simulink model "fullbridge1ph_mosfet_model2"  (R2026a)
settings: Solver=VariableStepAuto  StopTime=simStopTime
undefined symbols (not defined in the file): deadSamples, fout, fsw, ModIndex, Rload, Ts_ctrl, Vg
libraries: fl_lib x31, nesl_utility x28, ee_lib x11, simulink x1
settings Model: Creator=walmy  LastModifiedBy=walmy
settings SimscapeCC: SimscapeNominalValues="[{\"value\":\"1\",\"unit\":\"A\"},{\"value\":\"1\",\"unit\":\"bar\"},{\"value\":\"1\",\"unit\":\"cm^2\"},{\"value\":\"1\",\"unit\":\"cm^3/s\"},{\"value\":\"1\",\"unit\":\"kJ/kg\"},{\"value\":\"1\",\"unit\":\"kW\"},{\"value\":\"1\",\"unit\":\"l\"},{\"value\":\"1\",\"unit\":\"N\"},{\"value\":\"1\",\"unit\":\"N*m\"},{\"value\":\"1\",\"unit\":\"V\"}]"  SimscapeLogType=none  SimscapeLogDataHistory=5000.0

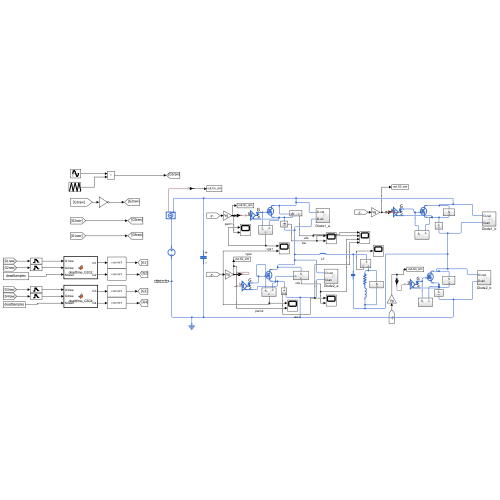
[thumbnail: Simulink's stored preview of the top-level diagram]
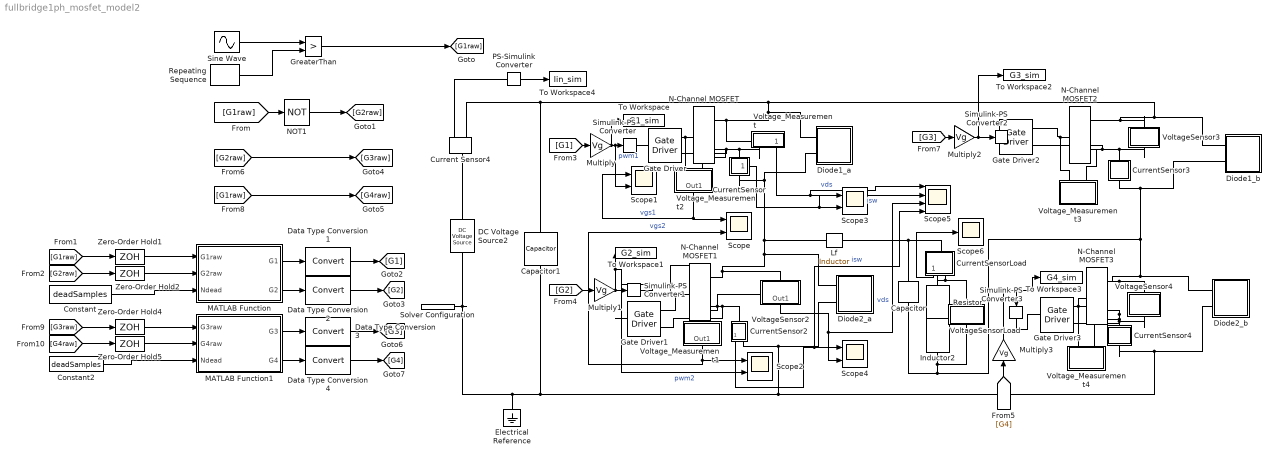
== system fullbridge1ph_mosfet_model2 ==
  Capacitor : fl_lib/Electrical/Electrical Elements/Capacitor  c=Cf F  r=0 Ohm  g=0 1/Ohm  i_specify=off  i_priority=None  i=0 A  i_nominal_specify=off  i_nominal_value=1  i_nominal_unit=A  v_specify=off  v_priority=High  v=0 V  v_nominal_specify=off  v_nominal_value=1  v_nominal_unit=V  vc_specify=on  vc_priority=High  vc=1 V  vc_nominal_specify=off  vc_nominal_value=1  vc_nominal_unit=V
  Capacitor1 : fl_lib/Electrical/Electrical Elements/Capacitor  c=Cdc F  r=0 Ohm  g=0 1/Ohm  i_specify=off  i_priority=None  i=0 A  i_nominal_specify=off  i_nominal_value=1  i_nominal_unit=A  v_specify=off  v_priority=High  v=Vdc V  v_nominal_specify=off  v_nominal_value=1  v_nominal_unit=V  vc_specify=on  vc_priority=High  vc=Vdc V  vc_nominal_specify=off  vc_nominal_value=1  vc_nominal_unit=V
  Constant : Constant  Value=deadSamples
  Constant2 : Constant  Value=deadSamples
  Current Sensor4 : fl_lib/Electrical/Electrical Sensors/Current Sensor
  CurrentSensor : Subsystem
      settings: PortSchema="{\"entries\":[{\"content\":{\"sides\":[{\"content\":{},\"type\":\"ConnectorPlacement.EquallySpacedRectSide\",\"uuid\":\"004a7a0d-f10a-4133-9832-9cba9dcbff9d\"},{\"content\":{\"connectorIds\":[\"Out1\"],\"side\":\"RIGHT\"},\"type\":\"ConnectorPlacement.EquallySpacedRectSide\",\"uuid\":\"56e408a5-c8db-4bda-b213-0e7e6169c543\"},{\"content\":{\"connectorIds\":[\"LConn1\"],\"side\":\"TOP\"},\"type\":\"ConnectorPlacement.EquallySpacedRectSide\",\"uuid\":\"d7e2417b-721d-4b46-aed4-551a16eadb47\"},{\"content\":{\"connectorIds\":[\"RConn1\"],\"side\":\"BOTTOM\"},\"type\":\"ConnectorPlacement.EquallySpacedRectSide\",\"uuid\":\"01b177b2-fa8e-4377-a3d9-543c30212534\"}]},\"type\":\"ConnectorPlacement.EquallySpacedConnector\",\"uuid\":\"4d702bd2-4ec5-4c77-8333-289479c4f2ec\"}],\"packageUris\":[\"http://schema.mathworks.com/mf0/Connector/R2020b\"],\"version\":\"1.0\"}"
  CurrentSensor2 : Subsystem
  CurrentSensor3 : Subsystem
  CurrentSensor4 : Subsystem
  CurrentSensorLoad : Subsystem
  DC Voltage Source2 : ee_lib/Additional Components/SPICE Sources/DC Voltage Source  DC=Vdc V
  Data Type Conversion{1..4} (4 alike) : DataTypeConversion  SaturateOnIntegerOverflow=off  RndMeth=Floor
  Diode1_a : Subsystem
  Diode1_b : Subsystem
  Diode2_a : Subsystem
  Diode2_b : Subsystem
  Electrical Reference : fl_lib/Electrical/Electrical Elements/Electrical Reference
  Gate Driver{,1..3} (4 alike) : ee_lib/Semiconductors & Converters/Gate Driver  port_option=ee.enum.controlport.ps  uHigh=2.0 V  uLow=0.8 V  uHighValue=0.7  uLowValue=0.3  vHigh=Vg V  vLow=-Vg V  tHigh=50 ns  tLow=50 ns  parameterization=ee.enum.semiconductors.gateDriverParam.outputImpedance  rHigh=Rg_on Ohm  rLow=Rg_off Ohm  tRise=20 ns  tFall=20 ns  cLoad=10 nF  ZonTime_specify=off  ZonTime_priority=None  ZonTime=0 s  ZoffTime_specify=off  ZoffTime_priority=None  ZoffTime=0 s
  GreaterThan : RelationalOperator  Operator=>  OutDataTypeStr=boolean  RndMeth=Simplest  InputSameDT=off
  Inductor2 : ee_lib/Passive/Inductor  l=Lload H  enable_L_tol=ee.enum.toleranceApplication.none  L_tol=20  tol_distribution=ee.enum.toleranceDistribution.uniform  nSigma=4  r=0 Ohm  g=1e-9 1/Ohm  enable_operating_limits=ee.enum.enable.no  operating_limit_action=ee.enum.passive.reportOpLim.warn  max_working_current=1 A  power_rating=1 W  i_L_specify=on  i_L_priority=Low  i_L=0 A  i_L_nominal_specify=off  i_L_nominal_value=1  i_L_nominal_unit=A
  Lf : ee_lib/Passive/Inductor  l=Lf H  enable_L_tol=ee.enum.toleranceApplication.none  L_tol=20  tol_distribution=ee.enum.toleranceDistribution.uniform  nSigma=4  r=0 Ohm  g=1e-9 1/Ohm  enable_operating_limits=ee.enum.enable.no  operating_limit_action=ee.enum.passive.reportOpLim.warn  max_working_current=1 A  power_rating=1 W  i_L_specify=on  i_L_priority=Low  i_L=0 A  i_L_nominal_specify=off  i_L_nominal_value=1  i_L_nominal_unit=A
  MATLAB Function : MATLAB Function  TreatAsAtomicUnit=on
  MATLAB Function1 : MATLAB Function  TreatAsAtomicUnit=on
  Multiply{,1..3} (4 alike) : Gain  Gain=Vg
  N-Channel MOSFET{,1..3} (4 alike) : ee_lib/Semiconductors & Converters/N-Channel MOSFET  paramTerminal=ee.enum.mosfet.numberOfTerminals.three  parameterization=ee.enum.mosfet.parameterization.datasheet  Beta=5.0 A/V^2  Rds=RdsOn Ohm  Id=Ids_RdsOn A  Vgs=Vgs_RdsOn V  Vth=Vth_sw V  Vth0=1.7 V  lam=0 1/V  gamma_vth=0.5 V^(1/2)  phib=0.5 V  Vth1=1.9071 V  Vbs1=-1 V  Vth2=2.066 V  Vbs2=-2 V  Tmeas=25 degC  Vgs_vec=[-1, -.5, 2, 3, 4, 5] V  Vds_vec=[0, 2, 4, 8, 12, 16, 20] V  Vbs_vec=[0, -4, -6, -12] V  T_vec=[25, 125] degC  Vth_vec=[.4, 1.2, 1.4, 1.45] V  Vth_mat=[.4, .35; 1.2, 1.15; 1.4, 1.35; 1.45, 1.4] V  Ids_mat=[0, 0, 0, 0, 0, 0, 0; 0, 0, 0, 0, 0, 0, 0; 0, .003, .0038, .0043, .0046, .0048, .0049; 0, .0055, .008, .009, .0095, .01, .0101; 0, .0115, .016, .018, .019, .0195, .02; 0, .0152, .0225, .0265, .028, .0295, .03] A  Ids_mat0=[0, 0, 0, 0, 0, 0, 0; 0, 0, 0, 0, 0, 0, 0; 0, .003, .0038, .0043, .0046, .0048, .0049; 0, .0055, .008, .009, .0095, .01, .0101; 0, .0115, .016, .018, .019, .0195, .02; 0, .0152, .0225, .0265, .028, .0295, .03] A  Ids_mat_3D=zeros(6, 7, 2) A  Ids_mat_3D0=zeros(6, 7, 2) A  IV_table_symmetry=ee.enum.mosfet.symmetricNIV.no  RS=0 Ohm  RD=0 Ohm  RB=0.001 Ohm  LeadRs=0 Ohm  LeadRd=0 Ohm  LeadRg=0 Ohm  LeadRb=0 Ohm  LS=0 nH  LD=0 nH  LG=0 nH  LB=0 nH  C_param=ee.enum.mosfet.capacitanceParam.fixedciss  C_GS=270 pF  C_GD=80 pF  C_GB=0 pF  C_DS=0 pF  C_iss=Ciss_sw_pF pF  C_rss=Crss_sw_pF pF  C_oss=Coss_sw_pF pF  C_iss_vec=[720, 700, 590, 470, 390, 310] pF  C_rss_vec=[450, 400, 300, 190, 95, 55] pF  C_oss_vec=[900, 810, 690, 420, 270, 170] pF  C_GS_vec=[270, 300, 290, 280, 295, 255] pF  C_GD_vec=[450, 400, 300, 190, 95, 55] pF  C_GB_vec=[270, 300, 290, 280, 295, 255] pF  C_Vgs_vec=0 V  C_DS_vec=[450, 410, 390, 230, 175, 115] pF  C_Vds_vec=[.1, .3, 1, 3, 10, 30] V  V_GS_for_cap_data=0 V  charge_linearity_param=ee.enum.mosfet.cgdLinearity.constant  C_OX=200 pF  V_C_OX=-0.5 V  charge_linearity_param_vgb=ee.enum.mosfet.cgbLinearity.instantly  charge_linearity_param_with_vgb=ee.enum.mosfet.cgbLinearityWithSeparateCgb.instantly  Di_param=ee.enum.mosfet.diodeParam.no  IsDiode=BodyDiodeIs A  Vbi=BodyDiodeVbi V  n=BodyDiodeN  Cj0Diode=BodyDiodeCj F  TT=BodyDiodeTT s  Tmeas_dio=25 degC  TableTypeNoT=ee.enum.mosfet.tableType.IfMat  TableType=ee.enum.diode.tableType.IfMat  IfVec=[.07, .12, .19, 1.75, 4.24, 7.32, 11.2] A  IfMat=[.07, .12, .19, 1.75, 4.24, 7.32, 11.2; .16, .3, .72, 2.14, 4.02, 6.35, 9.12] A  VfVecV=[.9, 1.15, 1.25, 1.5, 1.75, 2.17, 2.6, 2.85] V  VfMatV=[.9, 1.15, 1.25, 1.5, 1.75, 2.17, 2.6, 2.85; .58, .68, .75, 1.1, 1.38, 1.77, 2.27, 2.7] V  TjVec=[25, 125] degC  VfVec=[.5, .7, .9, 1.3, 1.7, 2.1, 2.5] V  IfVecV=[.1, .2, .5, 1, 2, 4, 7, 10] A  diode_Goff=1e-12 1/Ohm  prmDatasheet=ee.enum.temperatureParameterization.none  prmEquCoeff=ee.enum.temperatureParameterization.none  dVth_dT=-6 mV/K  dVth0_dT=-6 mV/K  Rds_T2=0.037 Ohm  BEXDatasheet=-1.5  BEXEquCoeff=-1.5  etaisDatasheet=3  etaisEquCoeff=3  Tmeas2=125 degC  etaisTabulated=3  TdeviceDatasheet=25 degC  TdeviceEquCoeff=25 degC  TdeviceTabulated=25 degC  i_g_specify=off  i_g_priority=None  i_g=0 A  i_g_nominal_specify=off  i_g_nominal_value=1  i_g_nominal_unit=A  i_d_specify=off  i_d_priority=None  i_d=0 A  i_d_nominal_specify=off  i_d_nominal_value=1  i_d_nominal_unit=A  i_b_specify=off  i_b_priority=None  i_b=0 A  i_b_nominal_specify=off  i_b_nominal_value=1  i_b_nominal_unit=A  voltage_gs_specify=off  voltage_gs_priority=None  voltage_gs=0 V  voltage_gs_nominal_specify=off  voltage_gs_nominal_value=1  voltage_gs_nominal_unit=V  voltage_ds_specify=off  voltage_ds_priority=None  voltage_ds=0 V  voltage_ds_nominal_specify=off  voltage_ds_nominal_value=1  voltage_ds_nominal_unit=V  voltage_bs_specify=off  voltage_bs_priority=None  voltage_bs=0 V  voltage_bs_nominal_specify=off  voltage_bs_nominal_value=1  voltage_bs_nominal_unit=V  v_Cgs_specify=off  v_Cgs_priority=High  v_Cgs=0 V  v_Cgs_nominal_specify=off  v_Cgs_nominal_value=1  v_Cgs_nominal_unit=V  v_Cds_specify=on  v_Cds_priority=Low  v_Cds=0 V  v_Cds_nominal_specify=off  v_Cds_nominal_value=1  v_Cds_nominal_unit=V  v_Cbs_specify=off  v_Cbs_priority=High  v_Cbs=0 V  v_Cbs_nominal_specify=off  v_Cbs_nominal_value=1  v_Cbs_nominal_unit=V  thermal_network_parameterization=ee.enum.thermalNetworkTopology.junctionCase  Rth=[0, 10] K/W  Rth_Cauer=[1, 3, 10] K/W  Rth_Foster=[.08, .14, .22, .16] K/W  thermal_mass_parameterization=ee.enum.thermalNetwork.timeconstant  thermal_mass=[0, 1] J/K  thermal_mass_Cauer=[.1, .3, 1] J/K  thermal_mass_Foster=[.001, .005, .05, .5] J/K  thermal_time_constant=[0, 10] s  thermal_time_constant_Cauer=[1, 3, 10] s  thermal_time_constant_Foster=[7e-05, .0007, .01, .08] s  thermal_mass_initial_temperatures=[25, 25] degC  thermal_mass_initial_temperatures_Cauer=[25, 25, 25] degC  Tvec_initial_Foster=[25, 25, 25, 25] degC  betaref=18 A/V^2  Vfbref=-1.1 V  gamma=3.5 V^(1/2)  phib2ref=1 V  thesatref=0.4 1/V  alpha=0  Vp=5e-2 V  thesrref=0 1/V  m=8  Tref=25 degC  Rsref=2e-3 Ohm  Rdref=0.17 Ohm  Rgref=8.4 Ohm  Rbref=2e-3 Ohm  Cox=1500 pF  Cgso=100 pF  Cgdo=14 pF  Isref=5.2e-13 A  Cj0=480 pF  Tprm=ee.enum.temperatureParameterization.none  etabet=1.3  Stvfb=5e-4 V/K  Stphib=-8.5e-4 V/K  etasat=1.04  etasr=0.65  etar=0.95  etais=3  Tsim=25 degC  Ig_specify=off  Ig_priority=None  Ig=0 A  Ig_nominal_specify=off  Ig_nominal_value=1  Ig_nominal_unit=nA  Ids_specify=off  Ids_priority=None  Ids=0 A  Ids_nominal_specify=off  Ids_nominal_value=1  Ids_nominal_unit=A  Ib_specify=off  Ib_priority=None  Ib=0 A  Ib_nominal_specify=off  Ib_nominal_value=1  Ib_nominal_unit=uA  V_gs_specify=off  V_gs_priority=None  V_gs=0 V  V_gs_nominal_specify=off  V_gs_nominal_value=1  V_gs_nominal_unit=V  V_ds_specify=off  V_ds_priority=None  V_ds=0 V  V_ds_nominal_specify=off  V_ds_nominal_value=1  V_ds_nominal_unit=V  V_bs_specify=off  V_bs_priority=None  V_bs=0 V  V_bs_nominal_specify=off  V_bs_nominal_value=1  V_bs_nominal_unit=V  QGoverCox_specify=off  QGoverCox_priority=None  QGoverCox=0 V  QGoverCox_nominal_specify=off  QGoverCox_nominal_value=1  QGoverCox_nominal_unit=V  QDoverCox_specify=off  QDoverCox_priority=None  QDoverCox=0 V  QDoverCox_nominal_specify=off  QDoverCox_nominal_value=1  QDoverCox_nominal_unit=V  QBoverCox_specify=off  QBoverCox_priority=None  QBoverCox=0 V  QBoverCox_nominal_specify=off  QBoverCox_nominal_value=1  QBoverCox_nominal_unit=V  T0=[25, 25] degC  T0_Cauer=[25, 25, 25] degC
  NOT1 : Logic  Operator=NOT  IconShape=distinctive  AllPortsSameDT=off  OutDataTypeStr=boolean
  PS-Simulink Converter : nesl_utility/PS-Simulink Converter  PhysicalDomain=network_engine_domain  SubClassName=ps_output  LeftPortType=input  RightPortType=output  PseudoPeriodic=off  Frequencies=[]  VectorFormat=inherit  Unit=inherit  AffineConversion=off
  Repeating Sequence : simulink/Sources/Repeating Sequence  rep_seq_t=[0 1/(2*fsw) 1/fsw]  rep_seq_y=[-1 1 -1]
  Resistor : fl_lib/Electrical/Electrical Elements/Resistor  R=Rload Ohm  i_specify=off  i_priority=None  i=0 A  i_nominal_specify=off  i_nominal_value=1  i_nominal_unit=A  v_specify=off  v_priority=None  v=0 V  v_nominal_specify=off  v_nominal_value=1  v_nominal_unit=V
  Scope{,1..4} (5 alike) : Scope  NumInputPorts=2
      Scope settings: ActiveDisplayYMinimum=-1.8442714573243091  ActiveDisplayYMaximum=11.329599284020166  DataLoggingVariableName=ScopeData2
      Scope1 settings: ActiveDisplayYMinimum=-1.6421747300623222  ActiveDisplayYMaximum=11.343693671801418  DataLoggingVariableName=ScopeData3
      Scope2 settings: ActiveDisplayYMinimum=-1  ActiveDisplayYMaximum=1  DataLoggingVariableName=ScopeData4
      Scope3 settings: ActiveDisplayYMinimum=-18.171152475957115  ActiveDisplayYMaximum=421.06855498709  DataLoggingVariableName=ScopeData5
      Scope4 settings: ActiveDisplayYMinimum=-1  ActiveDisplayYMaximum=1  DataLoggingVariableName=ScopeData6
  Scope5 : Scope  NumInputPorts=4
      settings: ActiveDisplayYMinimum=-77.946677692025617  ActiveDisplayYMaximum=455.393739095461  DataLoggingVariableName=ScopeData7
  Scope6 : Scope
      settings: ActiveDisplayYMinimum=-11.968033507226483  ActiveDisplayYMaximum=12.230491562923556
  Simulink-PS Converter{,1..3} (4 alike) : nesl_utility/Simulink-PS Converter  PhysicalDomain=network_engine_domain  SubClassName=ps_input  LeftPortType=input  RightPortType=output  PseudoPeriodic=off  Frequencies=[]  NoiseDistribution=none  NoiseParameters=[]  Unit=1  AffineConversion=off  FilteringAndDerivatives=provide  SimscapeFilterOrder=1  InputFilterTimeConstant=0.001  UdotUserProvided=0
  Sine Wave : Sin  Amplitude=ModIndex  Frequency=2*pi*fout  SampleTime=0
  Solver Configuration : nesl_utility/Solver Configuration  PhysicalDomain=network_engine_domain  SubClassName=solver  LeftPortType=input  RightPortType=generic  Tones=[]  Harmonics=[]  SimulateNoise=off  Profile=off  UseLocalSampling=off  EnableSwitchedLinearOptims=on  FrequencyDomain=off  UseCCode=off  RelTol=0.001  AbsTol=0.001  MinStep=1e-09  ToWorkspace=off  RevertToSquareIcSolve=off  NumHomotopyIterations=100  PhasorMode=off  PhasorModeNumHarmonics=1  ConsistencySolver=NEWTON_XTOL_AFTER_FTOL  CanonicalOrdering=UNORDERED  OptimizeIntermediates=UNOPTIMIZED  IndexReductionMethod=DerivativeReplacement  DoDC=off  ResidualTolerance=1e-09  ConsistencyTolSource=GLOBAL  ConsistencyAbsTol=0.001  ConsistencyRelTol=0.001  ConsistencyTolFactor=0.001  UseLocalSolver=on  LocalSolverChoice=NE_BACKWARD_EULER_ADVANCER  ResolveIndetEquations=on  FunctionEvalNumThread=1  LocalSolverSampleTime=50e-09  DoFixedCost=off  MaxNonlinIter=3  MaxModeIter=2  ComputeImpulses=off  ImpulseIterations=2  LinearAlgebra=auto  LinearAlgebraNumThread=0  EquationFormulation=NE_TIME_EF  DelaysMemoryBudget=1024  AutomaticFiltering=on  FilteringTimeConstant=0.001  PartitionStorageMethod=AS_NEEDED  PartitionMemoryBudget=1024  PartitionMethod=ROBUST  MultibodyUseLocalSolver=off  MultibodyLocalSolverChoice=ODE1  MultibodyLocalSolverSampleTime=0.001
  To Workspace : ToWorkspace  VariableName=G1_sim  SaveFormat=Timeseries  SampleTime=-1
  To Workspace1 : ToWorkspace  VariableName=G2_sim  SaveFormat=Timeseries  SampleTime=-1
  To Workspace2 : ToWorkspace  VariableName=G3_sim  SaveFormat=Timeseries  SampleTime=-1
  To Workspace3 : ToWorkspace  VariableName=G4_sim  SaveFormat=Timeseries  SampleTime=-1
  To Workspace4 : ToWorkspace  VariableName=Iin_sim  SaveFormat=Timeseries  SampleTime=-1
  VoltageSensor2 : Subsystem
      settings: PortSchema="{\"entries\":[{\"content\":{\"sides\":[{\"content\":{\"connectorIds\":[\"LConn1\"]},\"type\":\"ConnectorPlacement.EquallySpacedRectSide\",\"uuid\":\"21f317c2-e9e3-4775-bc2b-f44589605b73\"},{\"content\":{\"connectorIds\":[\"Out1\"],\"side\":\"RIGHT\"},\"type\":\"ConnectorPlacement.EquallySpacedRectSide\",\"uuid\":\"b0a4b85f-57a9-4dd8-a5ef-f426b86bae19\"},{\"content\":{\"connectorIds\":[\"LConn2\"],\"side\":\"TOP\"},\"type\":\"ConnectorPlacement.EquallySpacedRectSide\",\"uuid\":\"154dd31c-2e34-446c-ad4e-468f30782d57\"}]},\"type\":\"ConnectorPlacement.EquallySpacedConnector\",\"uuid\":\"ce3d8c78-d9da-4da1-88e6-92c14a3c1d9d\"}],\"packageUris\":[\"http://schema.mathworks.com/mf0/Connector/R2020b\"],\"version\":\"1.0\"}"
  VoltageSensor3 : Subsystem
  VoltageSensor4 : Subsystem
  VoltageSensorLoad : Subsystem
  Voltage_Measurement : Subsystem
      settings: PortSchema="{\"entries\":[{\"content\":{\"sides\":[{\"content\":{},\"type\":\"ConnectorPlacement.EquallySpacedRectSide\",\"uuid\":\"05335a37-bb92-4dc1-a41e-097329ec8732\"},{\"content\":{\"connectorIds\":[\"RConn1\",\"Out1\"],\"side\":\"RIGHT\"},\"type\":\"ConnectorPlacement.EquallySpacedRectSide\",\"uuid\":\"ddc17991-7e8e-4870-a1a0-8b769323db05\"},{\"content\":{\"connectorIds\":[\"LConn1\"],\"side\":\"TOP\"},\"type\":\"ConnectorPlacement.EquallySpacedRectSide\",\"uuid\":\"7075b36f-b4e1-42ca-a61e-d199b225f25e\"}]},\"type\":\"ConnectorPlacement.EquallySpacedConnector\",\"uuid\":\"382df35e-8f74-4d81-944e-45ad513cff4b\"}],\"packageUris\":[\"http://schema.mathworks.com/mf0/Connector/R2020b\"],\"version\":\"1.0\"}"
  Voltage_Measurement1 : Subsystem
  Voltage_Measurement2 : Subsystem
  Voltage_Measurement3 : Subsystem
  Voltage_Measurement4 : Subsystem
  Zero-Order Hold{1..2,4..5} (4 alike) : ZeroOrderHold  SampleTime=Ts_ctrl
  wires:
  [G1raw] -> Zero-Order Hold1/1
  [G2raw] -> Zero-Order Hold2/1
  MATLAB Function/1(G1) -> Data Type Conversion1/1
  MATLAB Function/2(G2) -> Data Type Conversion2/1
  [G1] -> Multiply/1
  Multiply3/1 -> To Workspace3/1, Simulink-PS Converter3/1
  Multiply2/1 -> To Workspace2/1, Simulink-PS Converter2/1
  [G1raw] -> NOT1/1
  NOT1/1 -> [G2raw]
  GreaterThan/1 -> [G1raw]
  Sine Wave/1 -> GreaterThan/1
  Repeating Sequence/1 -> GreaterThan/2
  [G2] -> Multiply1/1
  [G3] -> Multiply2/1
  [G4] -> Multiply3/1
  Data Type Conversion1/1 -> [G1]
  Data Type Conversion2/1 -> [G2]
  [G2raw] -> [G3raw]
  [G1raw] -> [G4raw]
  Data Type Conversion4/1 -> [G4]
  Data Type Conversion3/1 -> [G3]
  MATLAB Function1/2(G4) -> Data Type Conversion4/1
  MATLAB Function1/1(G3) -> Data Type Conversion3/1
  Constant2/1 -> MATLAB Function1/3(Ndead)
  [G4raw] -> Zero-Order Hold5/1
  [G3raw] -> Zero-Order Hold4/1
  Multiply1/1 -> Scope2/2, To Workspace1/1, Simulink-PS Converter1/1  "pwm2"
  Multiply/1 -> To Workspace/1, Simulink-PS Converter/1, Scope1/2  "pwm1"
  Voltage_Measurement2/1(Out1) -> Scope/1, Scope1/1  "vgs1"
  Voltage_Measurement1/1(Out1) -> Scope2/1, Scope/2  "vgs2"
  Voltage_Measurement/1(Out1) -> Scope5/1, Scope3/1  "vds"
  CurrentSensor/1(Out1) -> Scope5/2, Scope3/2  "isw"
  CurrentSensor2/1(Out1) -> Scope5/4, Scope4/1  "isw"
  VoltageSensor2/1(Out1) -> Scope5/3, Scope4/2  "vds"
  CurrentSensorLoad/1(Out1) -> Scope6/1
  PS-Simulink Converter/1 -> To Workspace4/1
  Zero-Order Hold1/1 -> MATLAB Function/1(G1raw)
  Zero-Order Hold2/1 -> MATLAB Function/2(G2raw)
  Constant/1 -> MATLAB Function/3(Ndead)
  Zero-Order Hold4/1 -> MATLAB Function1/1(G3raw)
  Zero-Order Hold5/1 -> MATLAB Function1/2(G4raw)
  connections:
  CurrentSensor4/RConn1 -- Solver Configuration/RConn1 -- DC Voltage Source2/RConn1 -- Electrical Reference/LConn1 -- Capacitor1/RConn1 -- Diode2_a/LConn2 -- CurrentSensor2/RConn1 -- Diode2_b/LConn2
  Diode1_a/LConn1 -- Voltage_Measurement/LConn1 -- N-Channel MOSFET/RConn1 -- Current Sensor4/RConn2 -- Capacitor1/LConn1 -- VoltageSensor3/LConn1 -- N-Channel MOSFET2/RConn1 -- Diode1_b/LConn1
  N-Channel MOSFET/RConn2 -- Voltage_Measurement/RConn1 -- CurrentSensor/LConn1 -- Gate Driver/RConn2 -- Voltage_Measurement2/LConn2
  CurrentSensor2/LConn1 -- Voltage_Measurement1/LConn2 -- VoltageSensor2/LConn2 -- Gate Driver1/RConn2 -- N-Channel MOSFET1/RConn2
  Diode2_a/LConn1 -- Diode1_a/LConn2 -- CurrentSensor/RConn1 -- Lf/LConn1 -- VoltageSensor2/LConn1 -- N-Channel MOSFET1/RConn1
  CurrentSensor3/LConn1 -- Voltage_Measurement3/LConn2 -- Gate Driver2/RConn2 -- N-Channel MOSFET2/RConn2 -- VoltageSensor3/RConn1
  Inductor2/RConn1 -- CurrentSensor3/RConn1 -- Diode1_b/LConn2 -- VoltageSensor4/LConn1 -- N-Channel MOSFET3/RConn1 -- Diode2_b/LConn1 -- Capacitor/RConn1 -- VoltageSensorLoad/RConn1
  CurrentSensor4/LConn1 -- Gate Driver3/RConn2 -- VoltageSensor4/RConn1 -- Voltage_Measurement4/LConn2 -- N-Channel MOSFET3/RConn2
  Capacitor/LConn1 -- CurrentSensorLoad/LConn1 -- Lf/RConn1
  Resistor/LConn1 -- VoltageSensorLoad/LConn1 -- CurrentSensorLoad/RConn1
  Resistor/RConn1 -- Inductor2/LConn1
  Gate Driver/RConn1 -- Voltage_Measurement2/LConn1 -- N-Channel MOSFET/LConn1
  Simulink-PS Converter/RConn1 -- Gate Driver/LConn1
  Gate Driver1/LConn1 -- Simulink-PS Converter1/RConn1
  Gate Driver2/LConn1 -- Simulink-PS Converter2/RConn1
  Voltage_Measurement3/LConn1 -- Gate Driver2/RConn1 -- N-Channel MOSFET2/LConn1
  Simulink-PS Converter3/RConn1 -- Gate Driver3/LConn1
  Gate Driver3/RConn1 -- Voltage_Measurement4/LConn1 -- N-Channel MOSFET3/LConn1
  Current Sensor4/LConn1 -- DC Voltage Source2/LConn1
  PS-Simulink Converter/LConn1 -- Current Sensor4/RConn1
  Gate Driver1/RConn1 -- Voltage_Measurement1/LConn1 -- N-Channel MOSFET1/LConn1

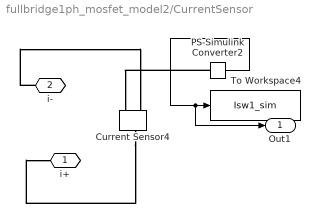
== system fullbridge1ph_mosfet_model2/CurrentSensor ==
  Current Sensor4 : fl_lib/Electrical/Electrical Sensors/Current Sensor
  PS-Simulink Converter2 : nesl_utility/PS-Simulink Converter  PhysicalDomain=network_engine_domain  SubClassName=ps_output  LeftPortType=input  RightPortType=output  PseudoPeriodic=off  Frequencies=[]  VectorFormat=inherit  Unit=inherit  AffineConversion=off
  To Workspace4 : ToWorkspace  VariableName=Isw1_sim  SaveFormat=Timeseries  SampleTime=-1
  i+ : PMIOPort  Side=Left
  i- : PMIOPort  Port=2  Side=Right
  Out1 : Outport
  wires:
  PS-Simulink Converter2/1 -> Out1/1, To Workspace4/1
  connections:
  Current Sensor4/LConn1 -- i+/RConn1
  PS-Simulink Converter2/LConn1 -- Current Sensor4/RConn1
  i-/RConn1 -- Current Sensor4/RConn2

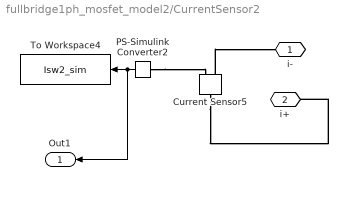
== system fullbridge1ph_mosfet_model2/CurrentSensor2 ==
  Current Sensor5 : fl_lib/Electrical/Electrical Sensors/Current Sensor
  PS-Simulink Converter2 : nesl_utility/PS-Simulink Converter  PhysicalDomain=network_engine_domain  SubClassName=ps_output  LeftPortType=input  RightPortType=output  PseudoPeriodic=off  Frequencies=[]  VectorFormat=inherit  Unit=inherit  AffineConversion=off
  To Workspace4 : ToWorkspace  VariableName=Isw2_sim  SaveFormat=Timeseries  SampleTime=-1
  i- : PMIOPort  Side=Right
  i+ : PMIOPort  Port=2  Side=Left
  Out1 : Outport
  wires:
  PS-Simulink Converter2/1 -> Out1/1, To Workspace4/1
  connections:
  PS-Simulink Converter2/LConn1 -- Current Sensor5/RConn1
  Current Sensor5/LConn1 -- i+/RConn1
  Current Sensor5/RConn2 -- i-/RConn1

== system fullbridge1ph_mosfet_model2/CurrentSensor3 ==
  Current Sensor2 : fl_lib/Electrical/Electrical Sensors/Current Sensor
  PS-Simulink Converter2 : nesl_utility/PS-Simulink Converter  PhysicalDomain=network_engine_domain  SubClassName=ps_output  LeftPortType=input  RightPortType=output  PseudoPeriodic=off  Frequencies=[]  VectorFormat=inherit  Unit=inherit  AffineConversion=off
  To Workspace4 : ToWorkspace  VariableName=Isw3_sim  SaveFormat=Timeseries  SampleTime=-1
  i- : PMIOPort  Side=Right
  i+ : PMIOPort  Port=2  Side=Left
  wires:
  PS-Simulink Converter2/1 -> To Workspace4/1
  connections:
  PS-Simulink Converter2/LConn1 -- Current Sensor2/RConn1
  i-/RConn1 -- Current Sensor2/RConn2
  Current Sensor2/LConn1 -- i+/RConn1

== system fullbridge1ph_mosfet_model2/CurrentSensor4 ==
  Current Sensor3 : fl_lib/Electrical/Electrical Sensors/Current Sensor
  PS-Simulink Converter2 : nesl_utility/PS-Simulink Converter  PhysicalDomain=network_engine_domain  SubClassName=ps_output  LeftPortType=input  RightPortType=output  PseudoPeriodic=off  Frequencies=[]  VectorFormat=inherit  Unit=inherit  AffineConversion=off
  To Workspace4 : ToWorkspace  VariableName=Isw4_sim  SaveFormat=Timeseries  SampleTime=-1
  i- : PMIOPort  Side=Right
  i+ : PMIOPort  Port=2  Side=Left
  wires:
  PS-Simulink Converter2/1 -> To Workspace4/1
  connections:
  PS-Simulink Converter2/LConn1 -- Current Sensor3/RConn1
  Current Sensor3/LConn1 -- i+/RConn1
  Current Sensor3/RConn2 -- i-/RConn1

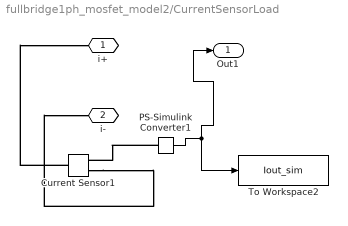
== system fullbridge1ph_mosfet_model2/CurrentSensorLoad ==
  Current Sensor1 : fl_lib/Electrical/Electrical Sensors/Current Sensor
  PS-Simulink Converter1 : nesl_utility/PS-Simulink Converter  PhysicalDomain=network_engine_domain  SubClassName=ps_output  LeftPortType=input  RightPortType=output  PseudoPeriodic=off  Frequencies=[]  VectorFormat=inherit  Unit=inherit  AffineConversion=off
  To Workspace2 : ToWorkspace  VariableName=Iout_sim  SaveFormat=Timeseries  SampleTime=-1
  i+ : PMIOPort  Side=Left
  i- : PMIOPort  Port=2  Side=Right
  Out1 : Outport
  wires:
  PS-Simulink Converter1/1 -> Out1/1, To Workspace2/1
  connections:
  PS-Simulink Converter1/LConn1 -- Current Sensor1/RConn1
  Current Sensor1/LConn1 -- i+/RConn1
  Current Sensor1/RConn2 -- i-/RConn1

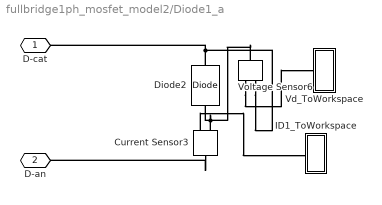
== system fullbridge1ph_mosfet_model2/Diode1_a ==
  Current Sensor3 : fl_lib/Electrical/Electrical Sensors/Current Sensor
  Diode2 : fl_lib/Electrical/Electrical Elements/Diode  Vf=Vf V  Ron=RonD Ohm  Goff=1e-8 1/Ohm  i_specify=off  i_priority=None  i=0 A  i_nominal_specify=off  i_nominal_value=1  i_nominal_unit=A  v_specify=off  v_priority=None  v=0 V  v_nominal_specify=off  v_nominal_value=1  v_nominal_unit=V
  ID1_ToWorkspace : Subsystem
      settings: PortSchema="{\"entries\":[{\"content\":{\"sides\":[{\"content\":{},\"type\":\"ConnectorPlacement.EquallySpacedRectSide\",\"uuid\":\"27aaa4b5-bd60-4d70-86e5-bc47b9bf8e53\"},{\"content\":{\"side\":\"RIGHT\"},\"type\":\"ConnectorPlacement.EquallySpacedRectSide\",\"uuid\":\"05934d8e-d6a5-4e4d-8439-d59dc6cd6ba8\"},{\"content\":{\"side\":\"TOP\"},\"type\":\"ConnectorPlacement.EquallySpacedRectSide\",\"uuid\":\"aced43fe-b59e-458d-8f58-35c4c9cdeb93\"},{\"content\":{\"connectorIds\":[\"RConn1\"],\"side\":\"BOTTOM\"},\"type\":\"ConnectorPlacement.EquallySpacedRectSide\",\"uuid\":\"aab3351d-4a00-4793-a207-44be8bae81b0\"}]},\"type\":\"ConnectorPlacement.EquallySpacedConnector\",\"uuid\":\"dcaf3857-8a00-4c3d-a0e7-096efad9ae0c\"}],\"packageUris\":[\"http://schema.mathworks.com/mf0/Connector/R2020b\"],\"version\":\"1.0\"}"
  Vd_ToWorkspace : Subsystem
      settings: PortSchema="{\"entries\":[{\"content\":{\"sides\":[{\"content\":{},\"type\":\"ConnectorPlacement.EquallySpacedRectSide\",\"uuid\":\"43f18de1-9718-4cbd-927a-ce7ec8f86ca1\"},{\"content\":{\"side\":\"RIGHT\"},\"type\":\"ConnectorPlacement.EquallySpacedRectSide\",\"uuid\":\"f671083a-78f6-4bee-900b-3feb52f79cdd\"},{\"content\":{\"side\":\"TOP\"},\"type\":\"ConnectorPlacement.EquallySpacedRectSide\",\"uuid\":\"024a9ce1-31bc-419f-b1bc-225b332881fb\"},{\"content\":{\"connectorIds\":[\"RConn1\"],\"side\":\"BOTTOM\"},\"type\":\"ConnectorPlacement.EquallySpacedRectSide\",\"uuid\":\"061c0d43-51f1-4fe9-9216-5b022de32a74\"}]},\"type\":\"ConnectorPlacement.EquallySpacedConnector\",\"uuid\":\"db5cc1c5-1d7d-4018-9977-3b4cf7cfcf03\"}],\"packageUris\":[\"http://schema.mathworks.com/mf0/Connector/R2020b\"],\"version\":\"1.0\"}"
  Voltage Sensor6 : fl_lib/Electrical/Electrical Sensors/Voltage Sensor
  D-cat : PMIOPort  Side=Left
  D-an : PMIOPort  Port=2  Side=Left
  connections:
  Current Sensor3/RConn2 -- Voltage Sensor6/LConn1 -- Diode2/LConn1
  Current Sensor3/RConn1 -- ID1_ToWorkspace/RConn1
  Diode2/RConn1 -- Voltage Sensor6/RConn2 -- D-cat/RConn1
  Voltage Sensor6/RConn1 -- Vd_ToWorkspace/RConn1
  Current Sensor3/LConn1 -- D-an/RConn1

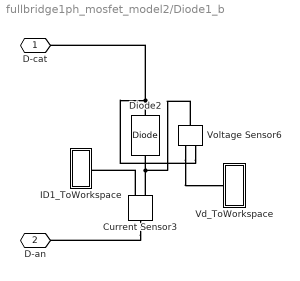
== system fullbridge1ph_mosfet_model2/Diode1_b ==
  Current Sensor3 : fl_lib/Electrical/Electrical Sensors/Current Sensor
  Diode2 : fl_lib/Electrical/Electrical Elements/Diode  Vf=Vf V  Ron=RonD Ohm  Goff=1e-8 1/Ohm  i_specify=off  i_priority=None  i=0 A  i_nominal_specify=off  i_nominal_value=1  i_nominal_unit=A  v_specify=off  v_priority=None  v=0 V  v_nominal_specify=off  v_nominal_value=1  v_nominal_unit=V
  ID1_ToWorkspace : Subsystem
      settings: PortSchema="{\"entries\":[{\"content\":{\"sides\":[{\"content\":{},\"type\":\"ConnectorPlacement.EquallySpacedRectSide\",\"uuid\":\"27aaa4b5-bd60-4d70-86e5-bc47b9bf8e53\"},{\"content\":{\"side\":\"RIGHT\"},\"type\":\"ConnectorPlacement.EquallySpacedRectSide\",\"uuid\":\"05934d8e-d6a5-4e4d-8439-d59dc6cd6ba8\"},{\"content\":{\"side\":\"TOP\"},\"type\":\"ConnectorPlacement.EquallySpacedRectSide\",\"uuid\":\"aced43fe-b59e-458d-8f58-35c4c9cdeb93\"},{\"content\":{\"connectorIds\":[\"RConn1\"],\"side\":\"BOTTOM\"},\"type\":\"ConnectorPlacement.EquallySpacedRectSide\",\"uuid\":\"aab3351d-4a00-4793-a207-44be8bae81b0\"}]},\"type\":\"ConnectorPlacement.EquallySpacedConnector\",\"uuid\":\"dcaf3857-8a00-4c3d-a0e7-096efad9ae0c\"}],\"packageUris\":[\"http://schema.mathworks.com/mf0/Connector/R2020b\"],\"version\":\"1.0\"}"
  Vd_ToWorkspace : Subsystem
      settings: PortSchema="{\"entries\":[{\"content\":{\"sides\":[{\"content\":{},\"type\":\"ConnectorPlacement.EquallySpacedRectSide\",\"uuid\":\"43f18de1-9718-4cbd-927a-ce7ec8f86ca1\"},{\"content\":{\"side\":\"RIGHT\"},\"type\":\"ConnectorPlacement.EquallySpacedRectSide\",\"uuid\":\"f671083a-78f6-4bee-900b-3feb52f79cdd\"},{\"content\":{\"side\":\"TOP\"},\"type\":\"ConnectorPlacement.EquallySpacedRectSide\",\"uuid\":\"024a9ce1-31bc-419f-b1bc-225b332881fb\"},{\"content\":{\"connectorIds\":[\"RConn1\"],\"side\":\"BOTTOM\"},\"type\":\"ConnectorPlacement.EquallySpacedRectSide\",\"uuid\":\"061c0d43-51f1-4fe9-9216-5b022de32a74\"}]},\"type\":\"ConnectorPlacement.EquallySpacedConnector\",\"uuid\":\"db5cc1c5-1d7d-4018-9977-3b4cf7cfcf03\"}],\"packageUris\":[\"http://schema.mathworks.com/mf0/Connector/R2020b\"],\"version\":\"1.0\"}"
  Voltage Sensor6 : fl_lib/Electrical/Electrical Sensors/Voltage Sensor
  D-cat : PMIOPort  Side=Left
  D-an : PMIOPort  Port=2  Side=Left
  connections:
  Current Sensor3/RConn2 -- Voltage Sensor6/LConn1 -- Diode2/LConn1
  Current Sensor3/RConn1 -- ID1_ToWorkspace/RConn1
  Diode2/RConn1 -- Voltage Sensor6/RConn2 -- D-cat/RConn1
  Voltage Sensor6/RConn1 -- Vd_ToWorkspace/RConn1
  Current Sensor3/LConn1 -- D-an/RConn1

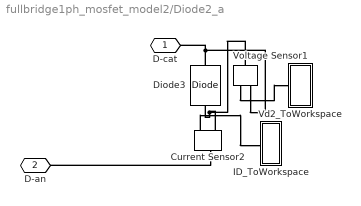
== system fullbridge1ph_mosfet_model2/Diode2_a ==
  Current Sensor2 : fl_lib/Electrical/Electrical Sensors/Current Sensor
  Diode3 : fl_lib/Electrical/Electrical Elements/Diode  Vf=Vf V  Ron=RonD Ohm  Goff=1e-8 1/Ohm  i_specify=off  i_priority=None  i=0 A  i_nominal_specify=off  i_nominal_value=1  i_nominal_unit=A  v_specify=off  v_priority=None  v=0 V  v_nominal_specify=off  v_nominal_value=1  v_nominal_unit=V
  ID_ToWorkspace : Subsystem
      settings: PortSchema="{\"entries\":[{\"content\":{\"sides\":[{\"content\":{},\"type\":\"ConnectorPlacement.EquallySpacedRectSide\",\"uuid\":\"5b175078-bf36-45f4-9d6d-54820150d16a\"},{\"content\":{\"side\":\"RIGHT\"},\"type\":\"ConnectorPlacement.EquallySpacedRectSide\",\"uuid\":\"3e3920a0-040e-4405-9234-56971fc67e62\"},{\"content\":{\"connectorIds\":[\"LConn1\"],\"side\":\"TOP\"},\"type\":\"ConnectorPlacement.EquallySpacedRectSide\",\"uuid\":\"d1eeb1f1-e8ae-4d22-bde1-4e1f65563d0c\"}]},\"type\":\"ConnectorPlacement.EquallySpacedConnector\",\"uuid\":\"fd63cd4a-cbe3-4add-a632-837285ffcc78\"}],\"packageUris\":[\"http://schema.mathworks.com/mf0/Connector/R2020b\"],\"version\":\"1.0\"}"
  Vd2_ToWorkspace : Subsystem
  Voltage Sensor1 : fl_lib/Electrical/Electrical Sensors/Voltage Sensor
  D-cat : PMIOPort  Side=Left
  D-an : PMIOPort  Port=2  Side=Left
  connections:
  Diode3/RConn1 -- Voltage Sensor1/RConn2 -- D-cat/RConn1
  Voltage Sensor1/RConn1 -- Vd2_ToWorkspace/LConn1
  Current Sensor2/RConn2 -- Voltage Sensor1/LConn1 -- Diode3/LConn1
  Current Sensor2/LConn1 -- D-an/RConn1
  Current Sensor2/RConn1 -- ID_ToWorkspace/LConn1

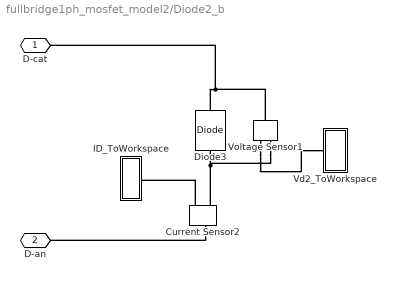
== system fullbridge1ph_mosfet_model2/Diode2_b ==
  Current Sensor2 : fl_lib/Electrical/Electrical Sensors/Current Sensor
  Diode3 : fl_lib/Electrical/Electrical Elements/Diode  Vf=Vf V  Ron=RonD Ohm  Goff=1e-8 1/Ohm  i_specify=off  i_priority=None  i=0 A  i_nominal_specify=off  i_nominal_value=1  i_nominal_unit=A  v_specify=off  v_priority=None  v=0 V  v_nominal_specify=off  v_nominal_value=1  v_nominal_unit=V
  ID_ToWorkspace : Subsystem
      settings: PortSchema="{\"entries\":[{\"content\":{\"sides\":[{\"content\":{},\"type\":\"ConnectorPlacement.EquallySpacedRectSide\",\"uuid\":\"5b175078-bf36-45f4-9d6d-54820150d16a\"},{\"content\":{\"side\":\"RIGHT\"},\"type\":\"ConnectorPlacement.EquallySpacedRectSide\",\"uuid\":\"3e3920a0-040e-4405-9234-56971fc67e62\"},{\"content\":{\"connectorIds\":[\"LConn1\"],\"side\":\"TOP\"},\"type\":\"ConnectorPlacement.EquallySpacedRectSide\",\"uuid\":\"d1eeb1f1-e8ae-4d22-bde1-4e1f65563d0c\"}]},\"type\":\"ConnectorPlacement.EquallySpacedConnector\",\"uuid\":\"fd63cd4a-cbe3-4add-a632-837285ffcc78\"}],\"packageUris\":[\"http://schema.mathworks.com/mf0/Connector/R2020b\"],\"version\":\"1.0\"}"
  Vd2_ToWorkspace : Subsystem
  Voltage Sensor1 : fl_lib/Electrical/Electrical Sensors/Voltage Sensor
  D-cat : PMIOPort  Side=Left
  D-an : PMIOPort  Port=2  Side=Left
  connections:
  Voltage Sensor1/LConn1 -- Diode3/RConn1 -- D-cat/RConn1
  Voltage Sensor1/RConn1 -- Vd2_ToWorkspace/LConn1
  Voltage Sensor1/RConn2 -- Current Sensor2/RConn2 -- Diode3/LConn1
  Current Sensor2/LConn1 -- D-an/RConn1
  Current Sensor2/RConn1 -- ID_ToWorkspace/LConn1

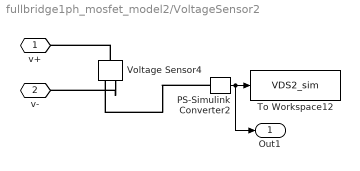
== system fullbridge1ph_mosfet_model2/VoltageSensor2 ==
  PS-Simulink Converter2 : nesl_utility/PS-Simulink Converter  PhysicalDomain=network_engine_domain  SubClassName=ps_output  LeftPortType=input  RightPortType=output  PseudoPeriodic=off  Frequencies=[]  VectorFormat=inherit  Unit=inherit  AffineConversion=off
  To Workspace12 : ToWorkspace  VariableName=VDS2_sim  SaveFormat=Timeseries  SampleTime=-1
  Voltage Sensor4 : fl_lib/Electrical/Electrical Sensors/Voltage Sensor
  v+ : PMIOPort  Side=Left
  v- : PMIOPort  Port=2  Side=Left
  Out1 : Outport
  wires:
  PS-Simulink Converter2/1 -> Out1/1, To Workspace12/1
  connections:
  PS-Simulink Converter2/LConn1 -- Voltage Sensor4/RConn1
  Voltage Sensor4/LConn1 -- v+/RConn1
  Voltage Sensor4/RConn2 -- v-/RConn1

== system fullbridge1ph_mosfet_model2/VoltageSensor3 ==
  PS-Simulink Converter1 : nesl_utility/PS-Simulink Converter  PhysicalDomain=network_engine_domain  SubClassName=ps_output  LeftPortType=input  RightPortType=output  PseudoPeriodic=off  Frequencies=[]  VectorFormat=inherit  Unit=inherit  AffineConversion=off
  To Workspace12 : ToWorkspace  VariableName=VDS3_sim  SaveFormat=Timeseries  SampleTime=-1
  Voltage Sensor1 : fl_lib/Electrical/Electrical Sensors/Voltage Sensor
  v+ : PMIOPort  Side=Left
  v- : PMIOPort  Port=2  Side=Right
  wires:
  PS-Simulink Converter1/1 -> To Workspace12/1
  connections:
  Voltage Sensor1/LConn1 -- v+/RConn1
  PS-Simulink Converter1/LConn1 -- Voltage Sensor1/RConn1
  Voltage Sensor1/RConn2 -- v-/RConn1

== system fullbridge1ph_mosfet_model2/VoltageSensor4 ==
  PS-Simulink Converter2 : nesl_utility/PS-Simulink Converter  PhysicalDomain=network_engine_domain  SubClassName=ps_output  LeftPortType=input  RightPortType=output  PseudoPeriodic=off  Frequencies=[]  VectorFormat=inherit  Unit=inherit  AffineConversion=off
  To Workspace12 : ToWorkspace  VariableName=VDS4_sim  SaveFormat=Timeseries  SampleTime=-1
  Voltage Sensor5 : fl_lib/Electrical/Electrical Sensors/Voltage Sensor
  v+ : PMIOPort  Side=Left
  v- : PMIOPort  Port=2  Side=Right
  wires:
  PS-Simulink Converter2/1 -> To Workspace12/1
  connections:
  PS-Simulink Converter2/LConn1 -- Voltage Sensor5/RConn1
  Voltage Sensor5/LConn1 -- v+/RConn1
  Voltage Sensor5/RConn2 -- v-/RConn1

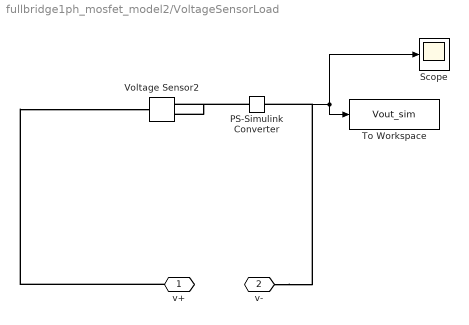
== system fullbridge1ph_mosfet_model2/VoltageSensorLoad ==
  PS-Simulink Converter : nesl_utility/PS-Simulink Converter  PhysicalDomain=network_engine_domain  SubClassName=ps_output  LeftPortType=input  RightPortType=output  PseudoPeriodic=off  Frequencies=[]  VectorFormat=inherit  Unit=inherit  AffineConversion=off
  Scope : Scope
      settings: ActiveDisplayYMinimum=-502.94177355107587  ActiveDisplayYMaximum=502.94249922447426
  To Workspace : ToWorkspace  VariableName=Vout_sim  SaveFormat=Timeseries  SampleTime=-1
  Voltage Sensor2 : fl_lib/Electrical/Electrical Sensors/Voltage Sensor
  v+ : PMIOPort  Side=Left
  v- : PMIOPort  Port=2  Side=Right
  wires:
  PS-Simulink Converter/1 -> Scope/1, To Workspace/1
  connections:
  PS-Simulink Converter/LConn1 -- Voltage Sensor2/RConn1
  v+/RConn1 -- Voltage Sensor2/LConn1
  v-/RConn1 -- Voltage Sensor2/RConn2

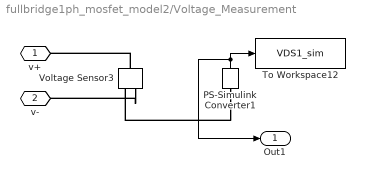
== system fullbridge1ph_mosfet_model2/Voltage_Measurement ==
  PS-Simulink Converter1 : nesl_utility/PS-Simulink Converter  PhysicalDomain=network_engine_domain  SubClassName=ps_output  LeftPortType=input  RightPortType=output  PseudoPeriodic=off  Frequencies=[]  VectorFormat=inherit  Unit=inherit  AffineConversion=off
  To Workspace12 : ToWorkspace  VariableName=VDS1_sim  SaveFormat=Timeseries  SampleTime=-1
  Voltage Sensor3 : fl_lib/Electrical/Electrical Sensors/Voltage Sensor
  v+ : PMIOPort  Side=Left
  v- : PMIOPort  Port=2  Side=Right
  Out1 : Outport
  wires:
  PS-Simulink Converter1/1 -> Out1/1, To Workspace12/1
  connections:
  Voltage Sensor3/LConn1 -- v+/RConn1
  PS-Simulink Converter1/LConn1 -- Voltage Sensor3/RConn1
  Voltage Sensor3/RConn2 -- v-/RConn1

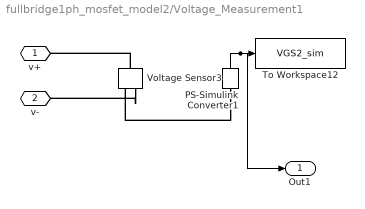
== system fullbridge1ph_mosfet_model2/Voltage_Measurement1 ==
  PS-Simulink Converter1 : nesl_utility/PS-Simulink Converter  PhysicalDomain=network_engine_domain  SubClassName=ps_output  LeftPortType=input  RightPortType=output  PseudoPeriodic=off  Frequencies=[]  VectorFormat=inherit  Unit=inherit  AffineConversion=off
  To Workspace12 : ToWorkspace  VariableName=VGS2_sim  SaveFormat=Timeseries  SampleTime=-1
  Voltage Sensor3 : fl_lib/Electrical/Electrical Sensors/Voltage Sensor
  v+ : PMIOPort  Side=Left
  v- : PMIOPort  Port=2  Side=Left
  Out1 : Outport
  wires:
  PS-Simulink Converter1/1 -> Out1/1, To Workspace12/1
  connections:
  Voltage Sensor3/RConn2 -- v-/RConn1
  PS-Simulink Converter1/LConn1 -- Voltage Sensor3/RConn1
  Voltage Sensor3/LConn1 -- v+/RConn1

== system fullbridge1ph_mosfet_model2/Voltage_Measurement2 ==
  PS-Simulink Converter1 : nesl_utility/PS-Simulink Converter  PhysicalDomain=network_engine_domain  SubClassName=ps_output  LeftPortType=input  RightPortType=output  PseudoPeriodic=off  Frequencies=[]  VectorFormat=inherit  Unit=inherit  AffineConversion=off
  To Workspace12 : ToWorkspace  VariableName=VGS1_sim  SaveFormat=Timeseries  SampleTime=-1
  Voltage Sensor3 : fl_lib/Electrical/Electrical Sensors/Voltage Sensor
  v+ : PMIOPort  Side=Left
  v- : PMIOPort  Port=2  Side=Left
  Out1 : Outport
  wires:
  PS-Simulink Converter1/1 -> Out1/1, To Workspace12/1
  connections:
  Voltage Sensor3/RConn2 -- v-/RConn1
  PS-Simulink Converter1/LConn1 -- Voltage Sensor3/RConn1
  Voltage Sensor3/LConn1 -- v+/RConn1

== system fullbridge1ph_mosfet_model2/Voltage_Measurement3 ==
  PS-Simulink Converter1 : nesl_utility/PS-Simulink Converter  PhysicalDomain=network_engine_domain  SubClassName=ps_output  LeftPortType=input  RightPortType=output  PseudoPeriodic=off  Frequencies=[]  VectorFormat=inherit  Unit=inherit  AffineConversion=off
  To Workspace12 : ToWorkspace  VariableName=VGS3_sim  SaveFormat=Timeseries  SampleTime=-1
  Voltage Sensor3 : fl_lib/Electrical/Electrical Sensors/Voltage Sensor
  v+ : PMIOPort  Side=Left
  v- : PMIOPort  Port=2  Side=Left
  wires:
  PS-Simulink Converter1/1 -> To Workspace12/1
  connections:
  Voltage Sensor3/RConn2 -- v-/RConn1
  PS-Simulink Converter1/LConn1 -- Voltage Sensor3/RConn1
  Voltage Sensor3/LConn1 -- v+/RConn1

== system fullbridge1ph_mosfet_model2/Voltage_Measurement4 ==
  PS-Simulink Converter1 : nesl_utility/PS-Simulink Converter  PhysicalDomain=network_engine_domain  SubClassName=ps_output  LeftPortType=input  RightPortType=output  PseudoPeriodic=off  Frequencies=[]  VectorFormat=inherit  Unit=inherit  AffineConversion=off
  To Workspace12 : ToWorkspace  VariableName=VGS4_sim  SaveFormat=Timeseries  SampleTime=-1
  Voltage Sensor3 : fl_lib/Electrical/Electrical Sensors/Voltage Sensor
  v+ : PMIOPort  Side=Left
  v- : PMIOPort  Port=2  Side=Left
  wires:
  PS-Simulink Converter1/1 -> To Workspace12/1
  connections:
  Voltage Sensor3/RConn2 -- v-/RConn1
  PS-Simulink Converter1/LConn1 -- Voltage Sensor3/RConn1
  Voltage Sensor3/LConn1 -- v+/RConn1

== system fullbridge1ph_mosfet_model2/Diode1_a/ID1_ToWorkspace ==
  PS-Simulink Converter1 : nesl_utility/PS-Simulink Converter  PhysicalDomain=network_engine_domain  SubClassName=ps_output  LeftPortType=input  RightPortType=output  PseudoPeriodic=off  Frequencies=[]  VectorFormat=inherit  Unit=inherit  AffineConversion=off
  To Workspace6 : ToWorkspace  VariableName=ID1_sim  SaveFormat=Timeseries  SampleTime=-1
  Conn1 : PMIOPort  Side=Right
  wires:
  PS-Simulink Converter1/1 -> To Workspace6/1
  connections:
  PS-Simulink Converter1/LConn1 -- Conn1/RConn1

== system fullbridge1ph_mosfet_model2/Diode1_a/Vd_ToWorkspace ==
  PS-Simulink Converter5 : nesl_utility/PS-Simulink Converter  PhysicalDomain=network_engine_domain  SubClassName=ps_output  LeftPortType=input  RightPortType=output  PseudoPeriodic=off  Frequencies=[]  VectorFormat=inherit  Unit=inherit  AffineConversion=off
  To Workspace12 : ToWorkspace  VariableName=VD1_sim  SaveFormat=Timeseries  SampleTime=-1
  y : PMIOPort  Side=Right
  wires:
  PS-Simulink Converter5/1 -> To Workspace12/1
  connections:
  y/RConn1 -- PS-Simulink Converter5/LConn1

== system fullbridge1ph_mosfet_model2/Diode1_b/ID1_ToWorkspace ==
  PS-Simulink Converter1 : nesl_utility/PS-Simulink Converter  PhysicalDomain=network_engine_domain  SubClassName=ps_output  LeftPortType=input  RightPortType=output  PseudoPeriodic=off  Frequencies=[]  VectorFormat=inherit  Unit=inherit  AffineConversion=off
  To Workspace6 : ToWorkspace  VariableName=ID3_sim  SaveFormat=Timeseries  SampleTime=-1
  Conn1 : PMIOPort  Side=Right
  wires:
  PS-Simulink Converter1/1 -> To Workspace6/1
  connections:
  PS-Simulink Converter1/LConn1 -- Conn1/RConn1

== system fullbridge1ph_mosfet_model2/Diode1_b/Vd_ToWorkspace ==
  PS-Simulink Converter5 : nesl_utility/PS-Simulink Converter  PhysicalDomain=network_engine_domain  SubClassName=ps_output  LeftPortType=input  RightPortType=output  PseudoPeriodic=off  Frequencies=[]  VectorFormat=inherit  Unit=inherit  AffineConversion=off
  To Workspace12 : ToWorkspace  VariableName=VD3_sim  SaveFormat=Timeseries  SampleTime=-1
  y : PMIOPort  Side=Right
  wires:
  PS-Simulink Converter5/1 -> To Workspace12/1
  connections:
  y/RConn1 -- PS-Simulink Converter5/LConn1

== system fullbridge1ph_mosfet_model2/Diode2_a/ID_ToWorkspace ==
  PS-Simulink Converter8 : nesl_utility/PS-Simulink Converter  PhysicalDomain=network_engine_domain  SubClassName=ps_output  LeftPortType=input  RightPortType=output  PseudoPeriodic=off  Frequencies=[]  VectorFormat=inherit  Unit=inherit  AffineConversion=off
  To Workspace6 : ToWorkspace  VariableName=ID2_sim  SaveFormat=Timeseries  SampleTime=-1
  y : PMIOPort  Side=Left
  wires:
  PS-Simulink Converter8/1 -> To Workspace6/1
  connections:
  y/RConn1 -- PS-Simulink Converter8/LConn1

== system fullbridge1ph_mosfet_model2/Diode2_a/Vd2_ToWorkspace ==
  PS-Simulink Converter7 : nesl_utility/PS-Simulink Converter  PhysicalDomain=network_engine_domain  SubClassName=ps_output  LeftPortType=input  RightPortType=output  PseudoPeriodic=off  Frequencies=[]  VectorFormat=inherit  Unit=inherit  AffineConversion=off
  To Workspace12 : ToWorkspace  VariableName=VD2_sim  SaveFormat=Timeseries  SampleTime=-1
  u : PMIOPort  Side=Left
  wires:
  PS-Simulink Converter7/1 -> To Workspace12/1
  connections:
  u/RConn1 -- PS-Simulink Converter7/LConn1

== system fullbridge1ph_mosfet_model2/Diode2_b/ID_ToWorkspace ==
  PS-Simulink Converter8 : nesl_utility/PS-Simulink Converter  PhysicalDomain=network_engine_domain  SubClassName=ps_output  LeftPortType=input  RightPortType=output  PseudoPeriodic=off  Frequencies=[]  VectorFormat=inherit  Unit=inherit  AffineConversion=off
  To Workspace6 : ToWorkspace  VariableName=ID4_sim  SaveFormat=Timeseries  SampleTime=-1
  y : PMIOPort  Side=Left
  wires:
  PS-Simulink Converter8/1 -> To Workspace6/1
  connections:
  y/RConn1 -- PS-Simulink Converter8/LConn1

== system fullbridge1ph_mosfet_model2/Diode2_b/Vd2_ToWorkspace ==
  PS-Simulink Converter7 : nesl_utility/PS-Simulink Converter  PhysicalDomain=network_engine_domain  SubClassName=ps_output  LeftPortType=input  RightPortType=output  PseudoPeriodic=off  Frequencies=[]  VectorFormat=inherit  Unit=inherit  AffineConversion=off
  To Workspace12 : ToWorkspace  VariableName=VD4_sim  SaveFormat=Timeseries  SampleTime=-1
  u : PMIOPort  Side=Left
  wires:
  PS-Simulink Converter7/1 -> To Workspace12/1
  connections:
  u/RConn1 -- PS-Simulink Converter7/LConn1

== matlab function fullbridge1ph_mosfet_model2/MATLAB Function1 ==
  data: G3raw input; G3 output; G4raw input; Ndead input; G4 output
function [G3, G4] = deadtime_G3G4(G3raw, G4raw, Ndead)

persistent G3_state G4_state cnt3 cnt4

if isempty(G3_state)
    G3_state = false;
    G4_state = false;
    cnt3 = 0;
    cnt4 = 0;
end

G3raw = logical(G3raw);
G4raw = logical(G4raw);
Ndead = max(0, round(Ndead));

if G3raw && G4raw
    G3_state = false;
    G4_state = false;
    cnt3 = 0;
    cnt4 = 0;

elseif G3raw
    G4_state = false;
    cnt4 = 0;

    if cnt3 >= Ndead
        G3_state = true;
    else
        G3_state = false;
        cnt3 = cnt3 + 1;
    end

elseif G4raw
    G3_state = false;
    cnt3 = 0;

    if cnt4 >= Ndead
        G4_state = true;
    else
        G4_state = false;
        cnt4 = cnt4 + 1;
    end

else
    G3_state = false;
    G4_state = false;
    cnt3 = 0;
    cnt4 = 0;
end

G3 = G3_state;
G4 = G4_state;

end

== matlab function fullbridge1ph_mosfet_model2/MATLAB Function ==
  data: G1raw input; G1 output; G2raw input; Ndead input; G2 output
function [G1, G2] = deadtime_G1G2(G1raw, G2raw, Ndead)

persistent G1_state G2_state cnt1 cnt2

if isempty(G1_state)
    G1_state = false;
    G2_state = false;
    cnt1 = 0;
    cnt2 = 0;
end

G1raw = logical(G1raw);
G2raw = logical(G2raw);
Ndead = max(0, round(Ndead));

if G1raw && G2raw
    G1_state = false;
    G2_state = false;
    cnt1 = 0;
    cnt2 = 0;

elseif G1raw
    G2_state = false;
    cnt2 = 0;

    if cnt1 >= Ndead
        G1_state = true;
    else
        G1_state = false;
        cnt1 = cnt1 + 1;
    end

elseif G2raw
    G1_state = false;
    cnt1 = 0;

    if cnt2 >= Ndead
        G2_state = true;
    else
        G2_state = false;
        cnt2 = cnt2 + 1;
    end

else
    G1_state = false;
    G2_state = false;
    cnt1 = 0;
    cnt2 = 0;
end

G1 = G1_state;
G2 = G2_state;

end
